simulink subsystem "v2021_10_27_Gear"  (R2020b)
settings: Solver=VariableStepAuto  StartTime=0.0  StopTime=10.0  RelTol=1e-3
values from neighbouring files (symbols this model uses):
  coeffAttritoStatico = 0.7    [v2021_10_27_avvioSITL.m]
  costantiMagicFormula = [ 10 1.3 1 0.95 ]    [v2021_10_27_avvioSITL.m]
  limitAinf = -500    [v2021_10_27_avvioSITL.m]
  limitAup = 500    [v2021_10_27_avvioSITL.m]
  limitPinf = -500    [v2021_10_27_avvioSITL.m]
  limitPup = 500    [v2021_10_27_avvioSITL.m]
  massaRuotaAnteriore = m    [v2021_10_27_avvioSITL.m]
  massaRuotePosteriori = m    [v2021_10_27_avvioSITL.m]
  Zpista = 0    [v2021_10_27_avvioSITL.m]
libraries: sharedutil x12, vrlib x9, simulink x1
(part 2 of 2)

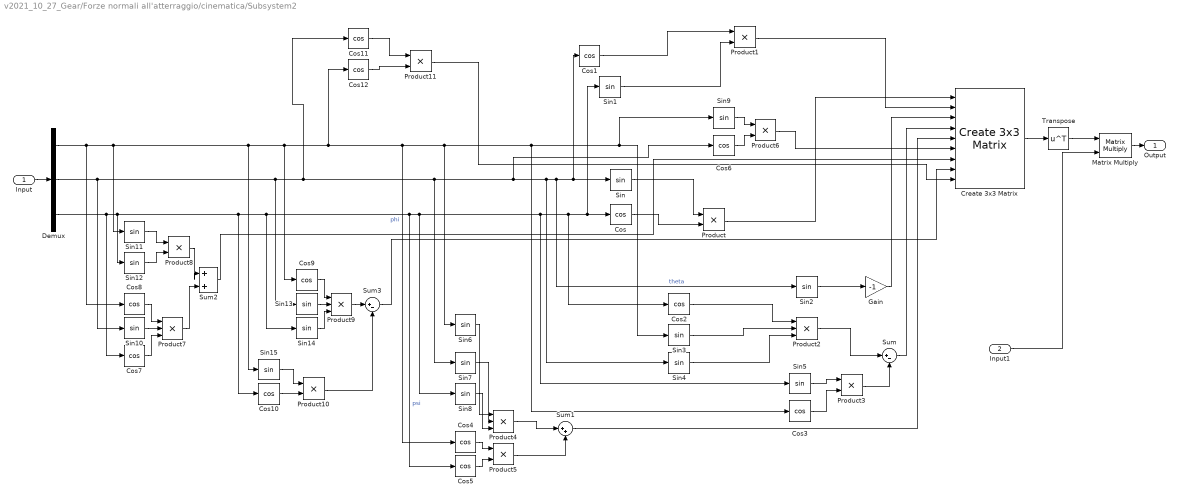
== system v2021_10_27_Gear/Forze normali all'atterraggio/cinematica/Subsystem2 ==
  Input : Inport
  Input1 : Inport  Port=2
  Cos{,1..12} (13 alike) : Trigonometry  Operator=cos
  Create 3x3 Matrix : sharedutil/Create 3x3 Matrix  aMode=aMode
  Demux : Demux  Outputs=3
  Gain : Gain  Gain=-1
  Matrix Multiply : Product  Multiplication=Matrix(*)
  Product{,1,3,5..6,8,10..11} (8 alike) : Product
  Product{2,4,7,9} (4 alike) : Product  Inputs=3
  Sin{,1..15} (16 alike) : Trigonometry
  Sum : Sum  Inputs=|+-
  Sum1 : Sum  Inputs=|++
  Sum2 : Sum  Inputs=|++
  Sum3 : Sum  Inputs=|+-
  Transpose : Math  Operator=transpose  SignedPower=on  SaturateOnIntegerOverflow=on
  Output : Outport  VectorParamsAs1DForOutWhenUnconnected=off
  wires:
  Transpose/1 -> Matrix Multiply/1
  Matrix Multiply/1 -> Output/1
  Input1/1 -> Matrix Multiply/2
  Create 3x3 Matrix/1 -> Transpose/1
  Product11/1 -> Create 3x3 Matrix/9
  Cos12/1 -> Product11/2
  Cos11/1 -> Product11/1
  Sum3/1 -> Create 3x3 Matrix/8
  Product10/1 -> Sum3/2
  Cos10/1 -> Product10/2
  Sin15/1 -> Product10/1
  Product9/1 -> Sum3/1
  Sin14/1 -> Product9/3
  Sin13/1 -> Product9/2
  Cos9/1 -> Product9/1
  Sum2/1 -> Create 3x3 Matrix/7
  Product8/1 -> Sum2/1
  Product7/1 -> Sum2/2
  Sin12/1 -> Product8/2
  Sin11/1 -> Product8/1
  Cos7/1 -> Product7/3
  Sin10/1 -> Product7/2
  Cos8/1 -> Product7/1
  Product6/1 -> Create 3x3 Matrix/6
  Cos6/1 -> Product6/2
  Sin9/1 -> Product6/1
  Sum1/1 -> Create 3x3 Matrix/5
  Product5/1 -> Sum1/2
  Product4/1 -> Sum1/1
  Cos5/1 -> Product5/2
  Cos4/1 -> Product5/1
  Sin8/1 -> Product4/3
  Sin7/1 -> Product4/2
  Sin6/1 -> Product4/1
  Sum/1 -> Create 3x3 Matrix/4
  Product3/1 -> Sum/2
  Cos3/1 -> Product3/2
  Sin5/1 -> Product3/1
  Sin4/1 -> Product2/3
  Cos2/1 -> Product2/1
  Product2/1 -> Sum/1
  Sin3/1 -> Product2/2
  Gain/1 -> Create 3x3 Matrix/3
  Demux/2 -> Sin/1, Cos1/1, Sin2/1, Sin4/1, Cos6/1, Sin7/1, Cos11/1, Sin13/1, Sin10/1  "theta"
  Sin2/1 -> Gain/1
  Product1/1 -> Create 3x3 Matrix/2
  Sin1/1 -> Product1/2
  Cos1/1 -> Product1/1
  Product/1 -> Create 3x3 Matrix/1
  Cos/1 -> Product/2
  Sin/1 -> Product/1
  Demux/3 -> Cos/1, Sin1/1, Cos2/1, Sin5/1, Sin8/1, Cos5/1, Sin14/1, Cos10/1, Sin12/1, Cos7/1  "psi"
  Demux/1 -> Sin11/1, Sin3/1, Sin9/1, Cos3/1, Sin6/1, Cos4/1, Cos12/1, Cos9/1, Sin15/1, Cos8/1  "phi"
  Input/1 -> Demux/1

== system v2021_10_27_Gear/Forze normali all'atterraggio1/Subsystem5/logica reset ==
  Input : Inport
  Constant : Constant  Value=0
  Pulse Generator : DiscretePulseGenerator  PulseType=Time based  Period=10  PulseWidth=0.1  PhaseDelay=2
  Switch : Switch  Criteria=u2 > Threshold
  Output : Outport
  wires:
  Switch/1 -> Output/1
  Constant/1 -> Switch/3
  Input/1 -> Switch/1
  Pulse Generator/1 -> Switch/2

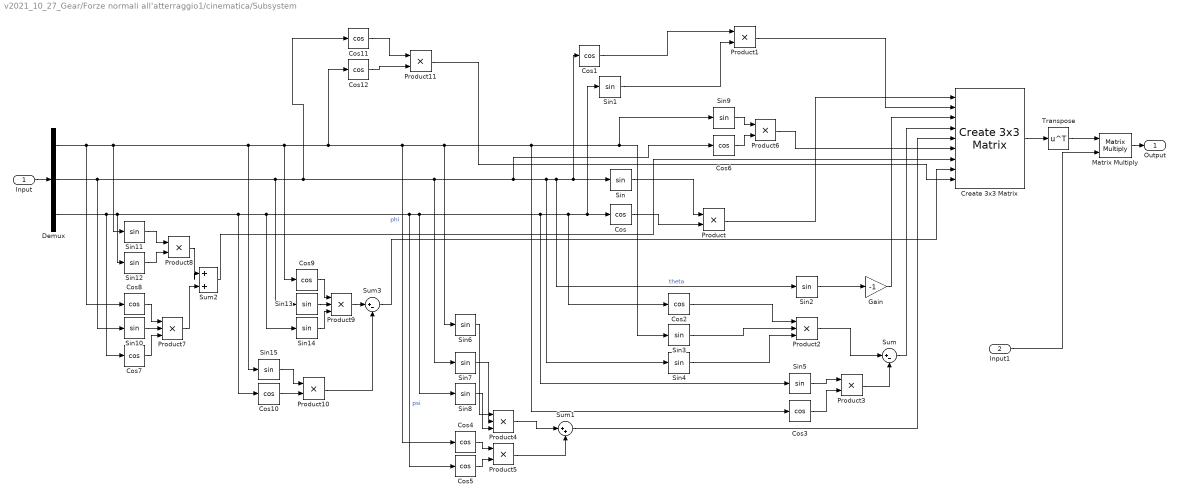
== system v2021_10_27_Gear/Forze normali all'atterraggio1/cinematica/Subsystem ==
  Input : Inport
  Input1 : Inport  Port=2
  Cos{,1..12} (13 alike) : Trigonometry  Operator=cos
  Create 3x3 Matrix : sharedutil/Create 3x3 Matrix  aMode=aMode
  Demux : Demux  Outputs=3
  Gain : Gain  Gain=-1
  Matrix Multiply : Product  Multiplication=Matrix(*)
  Product{,1,3,5..6,8,10..11} (8 alike) : Product
  Product{2,4,7,9} (4 alike) : Product  Inputs=3
  Sin{,1..15} (16 alike) : Trigonometry
  Sum : Sum  Inputs=|+-
  Sum1 : Sum  Inputs=|++
  Sum2 : Sum  Inputs=|++
  Sum3 : Sum  Inputs=|+-
  Transpose : Math  Operator=transpose  SignedPower=on  SaturateOnIntegerOverflow=on
  Output : Outport  VectorParamsAs1DForOutWhenUnconnected=off
  wires:
  Transpose/1 -> Matrix Multiply/1
  Matrix Multiply/1 -> Output/1
  Input1/1 -> Matrix Multiply/2
  Create 3x3 Matrix/1 -> Transpose/1
  Product11/1 -> Create 3x3 Matrix/9
  Cos12/1 -> Product11/2
  Cos11/1 -> Product11/1
  Sum3/1 -> Create 3x3 Matrix/8
  Product10/1 -> Sum3/2
  Cos10/1 -> Product10/2
  Sin15/1 -> Product10/1
  Product9/1 -> Sum3/1
  Sin14/1 -> Product9/3
  Sin13/1 -> Product9/2
  Cos9/1 -> Product9/1
  Sum2/1 -> Create 3x3 Matrix/7
  Product8/1 -> Sum2/1
  Product7/1 -> Sum2/2
  Sin12/1 -> Product8/2
  Sin11/1 -> Product8/1
  Cos7/1 -> Product7/3
  Sin10/1 -> Product7/2
  Cos8/1 -> Product7/1
  Product6/1 -> Create 3x3 Matrix/6
  Cos6/1 -> Product6/2
  Sin9/1 -> Product6/1
  Sum1/1 -> Create 3x3 Matrix/5
  Product5/1 -> Sum1/2
  Product4/1 -> Sum1/1
  Cos5/1 -> Product5/2
  Cos4/1 -> Product5/1
  Sin8/1 -> Product4/3
  Sin7/1 -> Product4/2
  Sin6/1 -> Product4/1
  Sum/1 -> Create 3x3 Matrix/4
  Product3/1 -> Sum/2
  Cos3/1 -> Product3/2
  Sin5/1 -> Product3/1
  Sin4/1 -> Product2/3
  Cos2/1 -> Product2/1
  Product2/1 -> Sum/1
  Sin3/1 -> Product2/2
  Gain/1 -> Create 3x3 Matrix/3
  Demux/2 -> Sin/1, Cos1/1, Sin2/1, Sin4/1, Cos6/1, Sin7/1, Cos11/1, Sin13/1, Sin10/1  "theta"
  Sin2/1 -> Gain/1
  Product1/1 -> Create 3x3 Matrix/2
  Sin1/1 -> Product1/2
  Cos1/1 -> Product1/1
  Product/1 -> Create 3x3 Matrix/1
  Cos/1 -> Product/2
  Sin/1 -> Product/1
  Demux/3 -> Cos/1, Sin1/1, Cos2/1, Sin5/1, Sin8/1, Cos5/1, Sin14/1, Cos10/1, Sin12/1, Cos7/1  "psi"
  Demux/1 -> Sin11/1, Sin3/1, Sin9/1, Cos3/1, Sin6/1, Cos4/1, Cos12/1, Cos9/1, Sin15/1, Cos8/1  "phi"
  Input/1 -> Demux/1

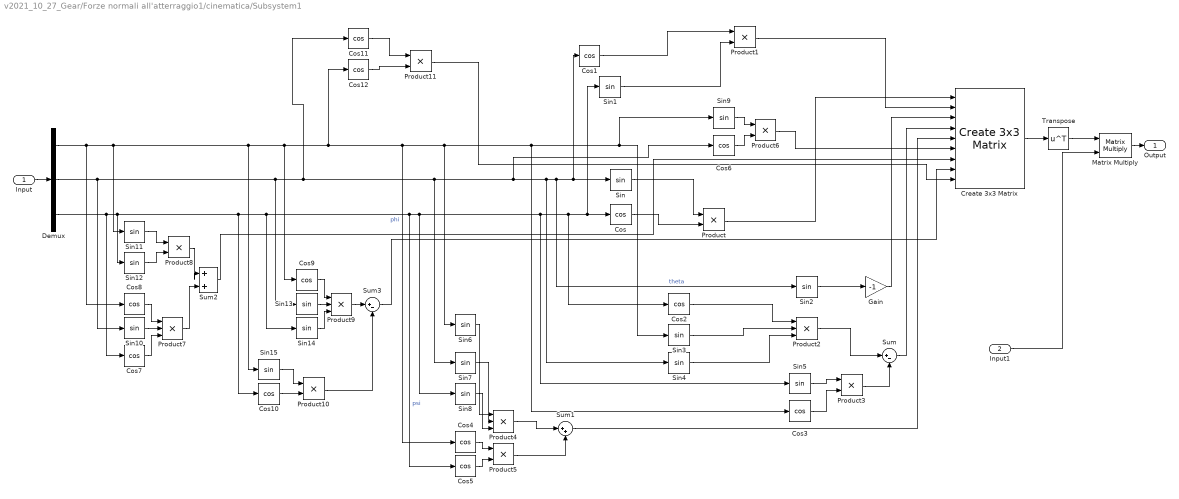
== system v2021_10_27_Gear/Forze normali all'atterraggio1/cinematica/Subsystem1 ==
  Input : Inport
  Input1 : Inport  Port=2
  Cos{,1..12} (13 alike) : Trigonometry  Operator=cos
  Create 3x3 Matrix : sharedutil/Create 3x3 Matrix  aMode=aMode
  Demux : Demux  Outputs=3
  Gain : Gain  Gain=-1
  Matrix Multiply : Product  Multiplication=Matrix(*)
  Product{,1,3,5..6,8,10..11} (8 alike) : Product
  Product{2,4,7,9} (4 alike) : Product  Inputs=3
  Sin{,1..15} (16 alike) : Trigonometry
  Sum : Sum  Inputs=|+-
  Sum1 : Sum  Inputs=|++
  Sum2 : Sum  Inputs=|++
  Sum3 : Sum  Inputs=|+-
  Transpose : Math  Operator=transpose  SignedPower=on  SaturateOnIntegerOverflow=on
  Output : Outport  VectorParamsAs1DForOutWhenUnconnected=off
  wires:
  Transpose/1 -> Matrix Multiply/1
  Matrix Multiply/1 -> Output/1
  Input1/1 -> Matrix Multiply/2
  Create 3x3 Matrix/1 -> Transpose/1
  Product11/1 -> Create 3x3 Matrix/9
  Cos12/1 -> Product11/2
  Cos11/1 -> Product11/1
  Sum3/1 -> Create 3x3 Matrix/8
  Product10/1 -> Sum3/2
  Cos10/1 -> Product10/2
  Sin15/1 -> Product10/1
  Product9/1 -> Sum3/1
  Sin14/1 -> Product9/3
  Sin13/1 -> Product9/2
  Cos9/1 -> Product9/1
  Sum2/1 -> Create 3x3 Matrix/7
  Product8/1 -> Sum2/1
  Product7/1 -> Sum2/2
  Sin12/1 -> Product8/2
  Sin11/1 -> Product8/1
  Cos7/1 -> Product7/3
  Sin10/1 -> Product7/2
  Cos8/1 -> Product7/1
  Product6/1 -> Create 3x3 Matrix/6
  Cos6/1 -> Product6/2
  Sin9/1 -> Product6/1
  Sum1/1 -> Create 3x3 Matrix/5
  Product5/1 -> Sum1/2
  Product4/1 -> Sum1/1
  Cos5/1 -> Product5/2
  Cos4/1 -> Product5/1
  Sin8/1 -> Product4/3
  Sin7/1 -> Product4/2
  Sin6/1 -> Product4/1
  Sum/1 -> Create 3x3 Matrix/4
  Product3/1 -> Sum/2
  Cos3/1 -> Product3/2
  Sin5/1 -> Product3/1
  Sin4/1 -> Product2/3
  Cos2/1 -> Product2/1
  Product2/1 -> Sum/1
  Sin3/1 -> Product2/2
  Gain/1 -> Create 3x3 Matrix/3
  Demux/2 -> Sin/1, Cos1/1, Sin2/1, Sin4/1, Cos6/1, Sin7/1, Cos11/1, Sin13/1, Sin10/1  "theta"
  Sin2/1 -> Gain/1
  Product1/1 -> Create 3x3 Matrix/2
  Sin1/1 -> Product1/2
  Cos1/1 -> Product1/1
  Product/1 -> Create 3x3 Matrix/1
  Cos/1 -> Product/2
  Sin/1 -> Product/1
  Demux/3 -> Cos/1, Sin1/1, Cos2/1, Sin5/1, Sin8/1, Cos5/1, Sin14/1, Cos10/1, Sin12/1, Cos7/1  "psi"
  Demux/1 -> Sin11/1, Sin3/1, Sin9/1, Cos3/1, Sin6/1, Cos4/1, Cos12/1, Cos9/1, Sin15/1, Cos8/1  "phi"
  Input/1 -> Demux/1

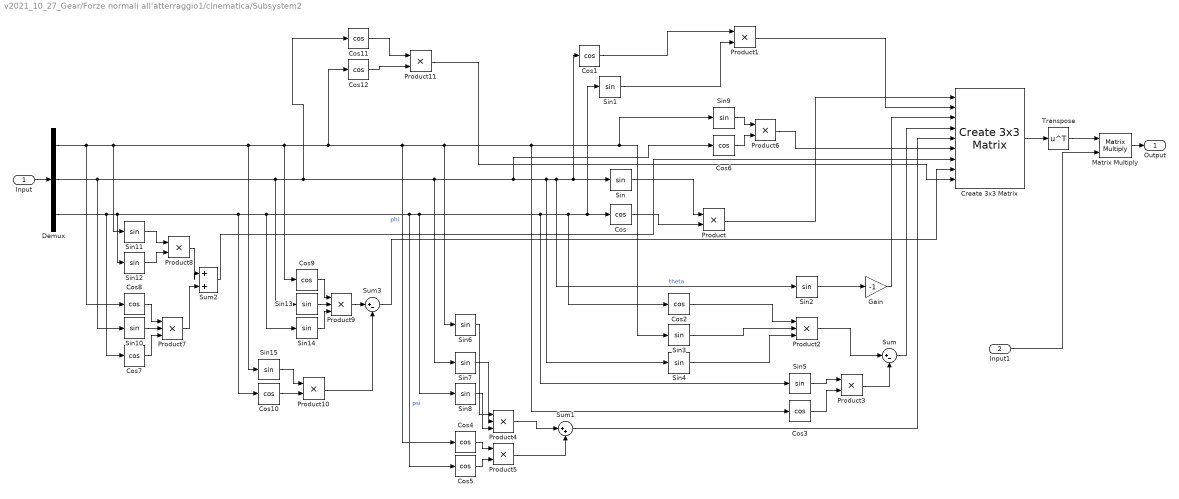
== system v2021_10_27_Gear/Forze normali all'atterraggio1/cinematica/Subsystem2 ==
  Input : Inport
  Input1 : Inport  Port=2
  Cos{,1..12} (13 alike) : Trigonometry  Operator=cos
  Create 3x3 Matrix : sharedutil/Create 3x3 Matrix  aMode=aMode
  Demux : Demux  Outputs=3
  Gain : Gain  Gain=-1
  Matrix Multiply : Product  Multiplication=Matrix(*)
  Product{,1,3,5..6,8,10..11} (8 alike) : Product
  Product{2,4,7,9} (4 alike) : Product  Inputs=3
  Sin{,1..15} (16 alike) : Trigonometry
  Sum : Sum  Inputs=|+-
  Sum1 : Sum  Inputs=|++
  Sum2 : Sum  Inputs=|++
  Sum3 : Sum  Inputs=|+-
  Transpose : Math  Operator=transpose  SignedPower=on  SaturateOnIntegerOverflow=on
  Output : Outport  VectorParamsAs1DForOutWhenUnconnected=off
  wires:
  Transpose/1 -> Matrix Multiply/1
  Matrix Multiply/1 -> Output/1
  Input1/1 -> Matrix Multiply/2
  Create 3x3 Matrix/1 -> Transpose/1
  Product11/1 -> Create 3x3 Matrix/9
  Cos12/1 -> Product11/2
  Cos11/1 -> Product11/1
  Sum3/1 -> Create 3x3 Matrix/8
  Product10/1 -> Sum3/2
  Cos10/1 -> Product10/2
  Sin15/1 -> Product10/1
  Product9/1 -> Sum3/1
  Sin14/1 -> Product9/3
  Sin13/1 -> Product9/2
  Cos9/1 -> Product9/1
  Sum2/1 -> Create 3x3 Matrix/7
  Product8/1 -> Sum2/1
  Product7/1 -> Sum2/2
  Sin12/1 -> Product8/2
  Sin11/1 -> Product8/1
  Cos7/1 -> Product7/3
  Sin10/1 -> Product7/2
  Cos8/1 -> Product7/1
  Product6/1 -> Create 3x3 Matrix/6
  Cos6/1 -> Product6/2
  Sin9/1 -> Product6/1
  Sum1/1 -> Create 3x3 Matrix/5
  Product5/1 -> Sum1/2
  Product4/1 -> Sum1/1
  Cos5/1 -> Product5/2
  Cos4/1 -> Product5/1
  Sin8/1 -> Product4/3
  Sin7/1 -> Product4/2
  Sin6/1 -> Product4/1
  Sum/1 -> Create 3x3 Matrix/4
  Product3/1 -> Sum/2
  Cos3/1 -> Product3/2
  Sin5/1 -> Product3/1
  Sin4/1 -> Product2/3
  Cos2/1 -> Product2/1
  Product2/1 -> Sum/1
  Sin3/1 -> Product2/2
  Gain/1 -> Create 3x3 Matrix/3
  Demux/2 -> Sin/1, Cos1/1, Sin2/1, Sin4/1, Cos6/1, Sin7/1, Cos11/1, Sin13/1, Sin10/1  "theta"
  Sin2/1 -> Gain/1
  Product1/1 -> Create 3x3 Matrix/2
  Sin1/1 -> Product1/2
  Cos1/1 -> Product1/1
  Product/1 -> Create 3x3 Matrix/1
  Cos/1 -> Product/2
  Sin/1 -> Product/1
  Demux/3 -> Cos/1, Sin1/1, Cos2/1, Sin5/1, Sin8/1, Cos5/1, Sin14/1, Cos10/1, Sin12/1, Cos7/1  "psi"
  Demux/1 -> Sin11/1, Sin3/1, Sin9/1, Cos3/1, Sin6/1, Cos4/1, Cos12/1, Cos9/1, Sin15/1, Cos8/1  "phi"
  Input/1 -> Demux/1

== system v2021_10_27_Gear/Forze normali all'atterraggio2/Subsystem5/logica reset ==
  Input : Inport
  Constant : Constant  Value=0
  Pulse Generator : DiscretePulseGenerator  PulseType=Time based  Period=10  PulseWidth=0.1  PhaseDelay=2
  Switch : Switch  Criteria=u2 > Threshold
  Output : Outport
  wires:
  Switch/1 -> Output/1
  Constant/1 -> Switch/3
  Input/1 -> Switch/1
  Pulse Generator/1 -> Switch/2

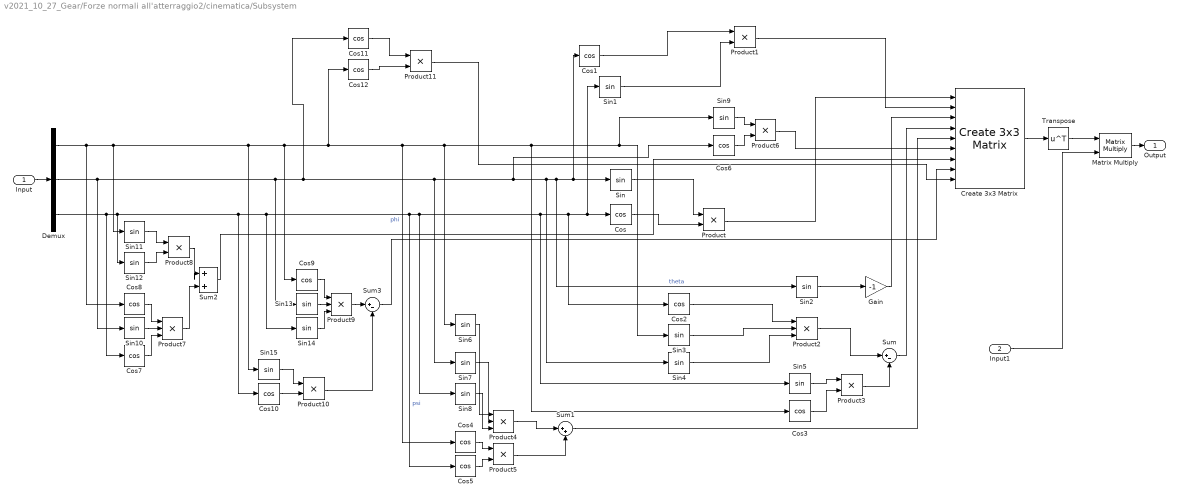
== system v2021_10_27_Gear/Forze normali all'atterraggio2/cinematica/Subsystem ==
  Input : Inport
  Input1 : Inport  Port=2
  Cos{,1..12} (13 alike) : Trigonometry  Operator=cos
  Create 3x3 Matrix : sharedutil/Create 3x3 Matrix  aMode=aMode
  Demux : Demux  Outputs=3
  Gain : Gain  Gain=-1
  Matrix Multiply : Product  Multiplication=Matrix(*)
  Product{,1,3,5..6,8,10..11} (8 alike) : Product
  Product{2,4,7,9} (4 alike) : Product  Inputs=3
  Sin{,1..15} (16 alike) : Trigonometry
  Sum : Sum  Inputs=|+-
  Sum1 : Sum  Inputs=|++
  Sum2 : Sum  Inputs=|++
  Sum3 : Sum  Inputs=|+-
  Transpose : Math  Operator=transpose  SignedPower=on  SaturateOnIntegerOverflow=on
  Output : Outport  VectorParamsAs1DForOutWhenUnconnected=off
  wires:
  Transpose/1 -> Matrix Multiply/1
  Matrix Multiply/1 -> Output/1
  Input1/1 -> Matrix Multiply/2
  Create 3x3 Matrix/1 -> Transpose/1
  Product11/1 -> Create 3x3 Matrix/9
  Cos12/1 -> Product11/2
  Cos11/1 -> Product11/1
  Sum3/1 -> Create 3x3 Matrix/8
  Product10/1 -> Sum3/2
  Cos10/1 -> Product10/2
  Sin15/1 -> Product10/1
  Product9/1 -> Sum3/1
  Sin14/1 -> Product9/3
  Sin13/1 -> Product9/2
  Cos9/1 -> Product9/1
  Sum2/1 -> Create 3x3 Matrix/7
  Product8/1 -> Sum2/1
  Product7/1 -> Sum2/2
  Sin12/1 -> Product8/2
  Sin11/1 -> Product8/1
  Cos7/1 -> Product7/3
  Sin10/1 -> Product7/2
  Cos8/1 -> Product7/1
  Product6/1 -> Create 3x3 Matrix/6
  Cos6/1 -> Product6/2
  Sin9/1 -> Product6/1
  Sum1/1 -> Create 3x3 Matrix/5
  Product5/1 -> Sum1/2
  Product4/1 -> Sum1/1
  Cos5/1 -> Product5/2
  Cos4/1 -> Product5/1
  Sin8/1 -> Product4/3
  Sin7/1 -> Product4/2
  Sin6/1 -> Product4/1
  Sum/1 -> Create 3x3 Matrix/4
  Product3/1 -> Sum/2
  Cos3/1 -> Product3/2
  Sin5/1 -> Product3/1
  Sin4/1 -> Product2/3
  Cos2/1 -> Product2/1
  Product2/1 -> Sum/1
  Sin3/1 -> Product2/2
  Gain/1 -> Create 3x3 Matrix/3
  Demux/2 -> Sin/1, Cos1/1, Sin2/1, Sin4/1, Cos6/1, Sin7/1, Cos11/1, Sin13/1, Sin10/1  "theta"
  Sin2/1 -> Gain/1
  Product1/1 -> Create 3x3 Matrix/2
  Sin1/1 -> Product1/2
  Cos1/1 -> Product1/1
  Product/1 -> Create 3x3 Matrix/1
  Cos/1 -> Product/2
  Sin/1 -> Product/1
  Demux/3 -> Cos/1, Sin1/1, Cos2/1, Sin5/1, Sin8/1, Cos5/1, Sin14/1, Cos10/1, Sin12/1, Cos7/1  "psi"
  Demux/1 -> Sin11/1, Sin3/1, Sin9/1, Cos3/1, Sin6/1, Cos4/1, Cos12/1, Cos9/1, Sin15/1, Cos8/1  "phi"
  Input/1 -> Demux/1

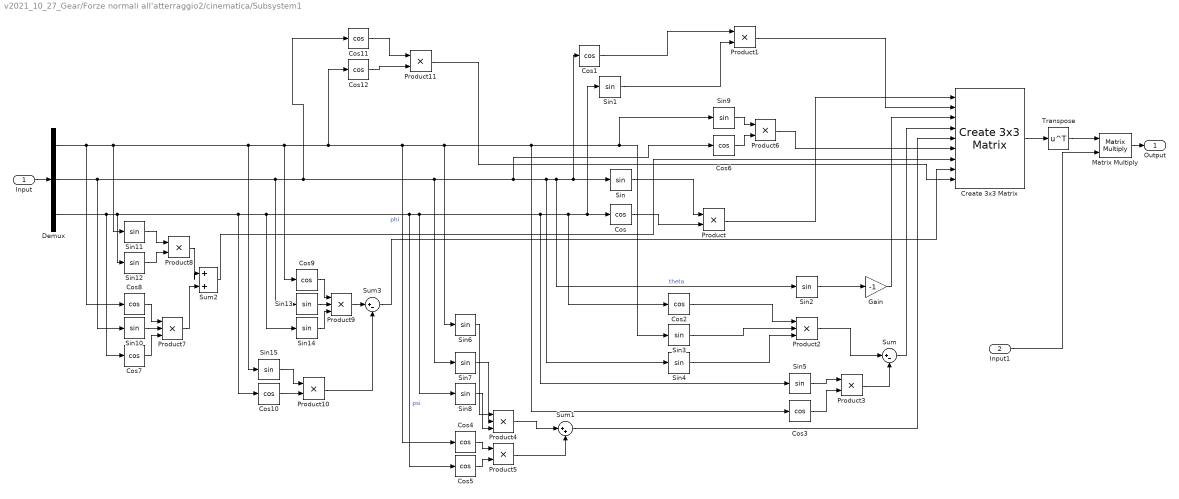
== system v2021_10_27_Gear/Forze normali all'atterraggio2/cinematica/Subsystem1 ==
  Input : Inport
  Input1 : Inport  Port=2
  Cos{,1..12} (13 alike) : Trigonometry  Operator=cos
  Create 3x3 Matrix : sharedutil/Create 3x3 Matrix  aMode=aMode
  Demux : Demux  Outputs=3
  Gain : Gain  Gain=-1
  Matrix Multiply : Product  Multiplication=Matrix(*)
  Product{,1,3,5..6,8,10..11} (8 alike) : Product
  Product{2,4,7,9} (4 alike) : Product  Inputs=3
  Sin{,1..15} (16 alike) : Trigonometry
  Sum : Sum  Inputs=|+-
  Sum1 : Sum  Inputs=|++
  Sum2 : Sum  Inputs=|++
  Sum3 : Sum  Inputs=|+-
  Transpose : Math  Operator=transpose  SignedPower=on  SaturateOnIntegerOverflow=on
  Output : Outport  VectorParamsAs1DForOutWhenUnconnected=off
  wires:
  Transpose/1 -> Matrix Multiply/1
  Matrix Multiply/1 -> Output/1
  Input1/1 -> Matrix Multiply/2
  Create 3x3 Matrix/1 -> Transpose/1
  Product11/1 -> Create 3x3 Matrix/9
  Cos12/1 -> Product11/2
  Cos11/1 -> Product11/1
  Sum3/1 -> Create 3x3 Matrix/8
  Product10/1 -> Sum3/2
  Cos10/1 -> Product10/2
  Sin15/1 -> Product10/1
  Product9/1 -> Sum3/1
  Sin14/1 -> Product9/3
  Sin13/1 -> Product9/2
  Cos9/1 -> Product9/1
  Sum2/1 -> Create 3x3 Matrix/7
  Product8/1 -> Sum2/1
  Product7/1 -> Sum2/2
  Sin12/1 -> Product8/2
  Sin11/1 -> Product8/1
  Cos7/1 -> Product7/3
  Sin10/1 -> Product7/2
  Cos8/1 -> Product7/1
  Product6/1 -> Create 3x3 Matrix/6
  Cos6/1 -> Product6/2
  Sin9/1 -> Product6/1
  Sum1/1 -> Create 3x3 Matrix/5
  Product5/1 -> Sum1/2
  Product4/1 -> Sum1/1
  Cos5/1 -> Product5/2
  Cos4/1 -> Product5/1
  Sin8/1 -> Product4/3
  Sin7/1 -> Product4/2
  Sin6/1 -> Product4/1
  Sum/1 -> Create 3x3 Matrix/4
  Product3/1 -> Sum/2
  Cos3/1 -> Product3/2
  Sin5/1 -> Product3/1
  Sin4/1 -> Product2/3
  Cos2/1 -> Product2/1
  Product2/1 -> Sum/1
  Sin3/1 -> Product2/2
  Gain/1 -> Create 3x3 Matrix/3
  Demux/2 -> Sin/1, Cos1/1, Sin2/1, Sin4/1, Cos6/1, Sin7/1, Cos11/1, Sin13/1, Sin10/1  "theta"
  Sin2/1 -> Gain/1
  Product1/1 -> Create 3x3 Matrix/2
  Sin1/1 -> Product1/2
  Cos1/1 -> Product1/1
  Product/1 -> Create 3x3 Matrix/1
  Cos/1 -> Product/2
  Sin/1 -> Product/1
  Demux/3 -> Cos/1, Sin1/1, Cos2/1, Sin5/1, Sin8/1, Cos5/1, Sin14/1, Cos10/1, Sin12/1, Cos7/1  "psi"
  Demux/1 -> Sin11/1, Sin3/1, Sin9/1, Cos3/1, Sin6/1, Cos4/1, Cos12/1, Cos9/1, Sin15/1, Cos8/1  "phi"
  Input/1 -> Demux/1

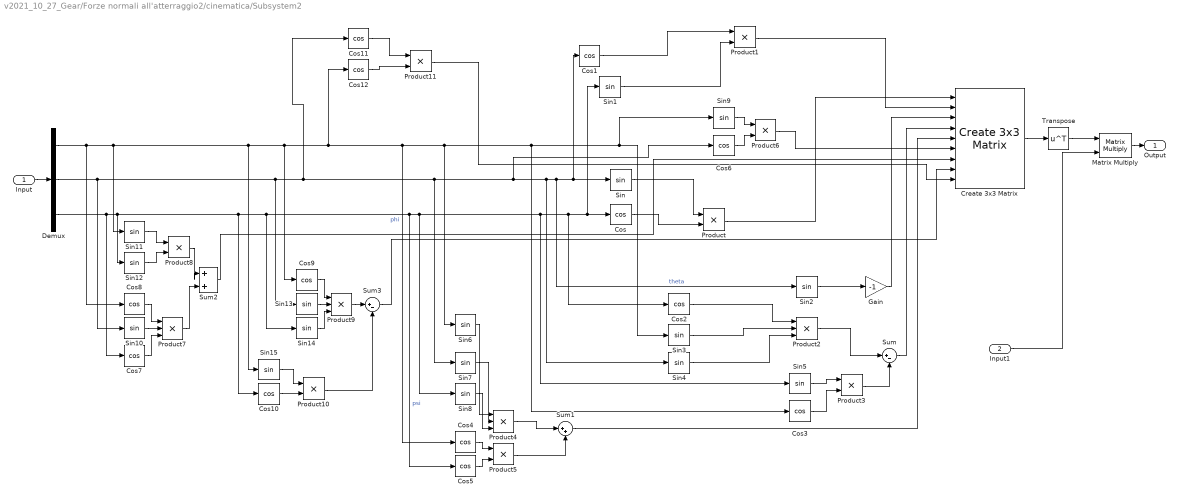
== system v2021_10_27_Gear/Forze normali all'atterraggio2/cinematica/Subsystem2 ==
  Input : Inport
  Input1 : Inport  Port=2
  Cos{,1..12} (13 alike) : Trigonometry  Operator=cos
  Create 3x3 Matrix : sharedutil/Create 3x3 Matrix  aMode=aMode
  Demux : Demux  Outputs=3
  Gain : Gain  Gain=-1
  Matrix Multiply : Product  Multiplication=Matrix(*)
  Product{,1,3,5..6,8,10..11} (8 alike) : Product
  Product{2,4,7,9} (4 alike) : Product  Inputs=3
  Sin{,1..15} (16 alike) : Trigonometry
  Sum : Sum  Inputs=|+-
  Sum1 : Sum  Inputs=|++
  Sum2 : Sum  Inputs=|++
  Sum3 : Sum  Inputs=|+-
  Transpose : Math  Operator=transpose  SignedPower=on  SaturateOnIntegerOverflow=on
  Output : Outport  VectorParamsAs1DForOutWhenUnconnected=off
  wires:
  Transpose/1 -> Matrix Multiply/1
  Matrix Multiply/1 -> Output/1
  Input1/1 -> Matrix Multiply/2
  Create 3x3 Matrix/1 -> Transpose/1
  Product11/1 -> Create 3x3 Matrix/9
  Cos12/1 -> Product11/2
  Cos11/1 -> Product11/1
  Sum3/1 -> Create 3x3 Matrix/8
  Product10/1 -> Sum3/2
  Cos10/1 -> Product10/2
  Sin15/1 -> Product10/1
  Product9/1 -> Sum3/1
  Sin14/1 -> Product9/3
  Sin13/1 -> Product9/2
  Cos9/1 -> Product9/1
  Sum2/1 -> Create 3x3 Matrix/7
  Product8/1 -> Sum2/1
  Product7/1 -> Sum2/2
  Sin12/1 -> Product8/2
  Sin11/1 -> Product8/1
  Cos7/1 -> Product7/3
  Sin10/1 -> Product7/2
  Cos8/1 -> Product7/1
  Product6/1 -> Create 3x3 Matrix/6
  Cos6/1 -> Product6/2
  Sin9/1 -> Product6/1
  Sum1/1 -> Create 3x3 Matrix/5
  Product5/1 -> Sum1/2
  Product4/1 -> Sum1/1
  Cos5/1 -> Product5/2
  Cos4/1 -> Product5/1
  Sin8/1 -> Product4/3
  Sin7/1 -> Product4/2
  Sin6/1 -> Product4/1
  Sum/1 -> Create 3x3 Matrix/4
  Product3/1 -> Sum/2
  Cos3/1 -> Product3/2
  Sin5/1 -> Product3/1
  Sin4/1 -> Product2/3
  Cos2/1 -> Product2/1
  Product2/1 -> Sum/1
  Sin3/1 -> Product2/2
  Gain/1 -> Create 3x3 Matrix/3
  Demux/2 -> Sin/1, Cos1/1, Sin2/1, Sin4/1, Cos6/1, Sin7/1, Cos11/1, Sin13/1, Sin10/1  "theta"
  Sin2/1 -> Gain/1
  Product1/1 -> Create 3x3 Matrix/2
  Sin1/1 -> Product1/2
  Cos1/1 -> Product1/1
  Product/1 -> Create 3x3 Matrix/1
  Cos/1 -> Product/2
  Sin/1 -> Product/1
  Demux/3 -> Cos/1, Sin1/1, Cos2/1, Sin5/1, Sin8/1, Cos5/1, Sin14/1, Cos10/1, Sin12/1, Cos7/1  "psi"
  Demux/1 -> Sin11/1, Sin3/1, Sin9/1, Cos3/1, Sin6/1, Cos4/1, Cos12/1, Cos9/1, Sin15/1, Cos8/1  "phi"
  Input/1 -> Demux/1

== matlab function v2021_10_27_Gear/Subsystem/MATLAB Function1 ==
  data: Fx output; B input; Fy output; C input; D input; E input; beta input; Fa input
function [Fx,Fy] = MacicFormula(B,C,D,E,beta,Fa)
%funzione matlab che calcola in modulo la Fy istantanea usando la magic 
%formula di Pacejka e poi calcola la Fx per differenza di vettori tra la Fa
%massima e la Fy calcolata
%se per caso |Fy|>0.5|Fa| si pone che Fy = Fa/2 per evitare problemi con la
%sqrt (non dovrebbe capitare mai).
Fy = -1*D*sin(C*atan(B*beta-E*(B*beta-atan(B*beta))));
if abs(Fy)>abs(Fa/2)
    Fy = -Fa/2;
end
Fx = 1*sqrt(Fa^2-Fy^2);

== matlab function v2021_10_27_Gear/Subsystem/MATLAB Function3 ==
  data: forzanormale input; forza_normale output
function forza_normale = contatto(forzanormale)
%questa funzione pone a 0 la forza normale se essa è minore di 0
if forzanormale > 0
    forza_normale = 0;
else
    forza_normale = forzanormale;
end

== matlab function v2021_10_27_Gear/Subsystem1/MATLAB Function1 ==
  data: Fx output; B input; Fy output; C input; D input; E input; beta input; Fa input
function [Fx,Fy] = MacicFormula(B,C,D,E,beta,Fa)
%funzione matlab che calcola in modulo la Fy istantanea usando la magic 
%formula di Pacejka e poi calcola la Fx per differenza di vettori tra la Fa
%massima e la Fy calcolata
%se per caso |Fy|>0.5|Fa| si pone che Fy = Fa/2 per evitare problemi con la
%sqrt (non dovrebbe capitare mai).
Fy = -1*D*sin(C*atan(B*beta-E*(B*beta-atan(B*beta))));
if abs(Fy)>abs(Fa/2)
    Fy = -Fa/2;
end
Fx = 1*sqrt(Fa^2-Fy^2);

== matlab function v2021_10_27_Gear/Subsystem1/MATLAB Function3 ==
  data: forzanormale input; forza_normale output
function forza_normale = contatto(forzanormale)
%questa funzione pone a 0 la forza normale se essa è minore di 0
if forzanormale > 0
    forza_normale = 0;
else
    forza_normale = forzanormale;
end

== matlab function v2021_10_27_Gear/Subsystem2/MATLAB Function1 ==
  data: Fx output; B input; Fy output; C input; D input; E input; beta input; Fa input
function [Fx,Fy] = MacicFormula(B,C,D,E,beta,Fa)
%funzione matlab che calcola in modulo la Fy istantanea usando la magic 
%formula di Pacejka e poi calcola la Fx per differenza di vettori tra la Fa
%massima e la Fy calcolata
%se per caso |Fy|>0.5|Fa| si pone che Fy = Fa/2 per evitare problemi con la
%sqrt (non dovrebbe capitare mai).
Fy = -1*D*sin(C*atan(B*beta-E*(B*beta-atan(B*beta))));
if abs(Fy)>abs(Fa/2)
    Fy = -Fa/2;
end
Fx = 1*sqrt(Fa^2-Fy^2);

== matlab function v2021_10_27_Gear/Subsystem2/MATLAB Function3 ==
  data: forzanormale input; forza_normale output
function forza_normale = contatto(forzanormale)
%questa funzione pone a 0 la forza normale se essa è maggiore di 0 (con
%riferimento agli assi corpo)
if forzanormale > 0
    forza_normale = 0;
else
    forza_normale = forzanormale;
end

== matlab function v2021_10_27_Gear/new_AL ==
  data: FNs input; Fza output; FNd input; FNa input; hant input; Fzps output; Fzpd output; hpostd input; hposts input; selector_AL input
function [Fza,Fzps,Fzpd] = forzenormaliatterraggio(FNs,FNd,FNa,hant,hpostd,hposts,selector_AL)

if  selector_AL==2 && hant>=-0.3925
    Fza=FNa;   
else
    Fza = 0;
end

if  selector_AL==2 && hpostd>=-0.3925
    Fzpd= FNd;
else
    Fzpd = 0;
end

if selector_AL==2 && hposts>=-0.3925
    Fzps= FNs;
else
    Fzps = 0;
end

== matlab function v2021_10_27_Gear/new_ATO ==
  data: Rmt input; Sbt input; MB input; FB input; Fza output; Fase_Ato input; FNs input; FNd input; FNa input; Fzps output; Fzpd output; clock input
function [Fza,Fzps,Fzpd] = forzenormalidecollo(Rmt,Sbt,MB,FB,Fase_Ato,FNs,FNd,FNa,clock)
Xa = Sbt(1);
Xp = Rmt(1);

if Fase_Ato == 4
         Fzps = 0;
         Fzpd = 0;
         Fza = 0;
elseif Fase_Ato == 3
    Fzps= FNs+(Xa*9.4*9.81)/(2*(Xa-Xp));
    Fzpd= FNd+(Xa*9.4*9.81)/(2*(Xa-Xp));
    Fza=0;
else
    Fzps= FNs+(Xa*9.4*9.81)/(2*(Xa-Xp));
    Fzpd= FNd+(Xa*9.4*9.81)/(2*(Xa-Xp));
    Fza = FNa+(-Xp*9.4*9.81)/(Xa-Xp);        
end
